simulink model "volt_mfile"  (R2019a)
settings: Solver=VariableStepAuto  StartTime=0.0  StopTime=5  RelTol=1e-3
settings Model: Creator=USER  LastModifiedBy=USER

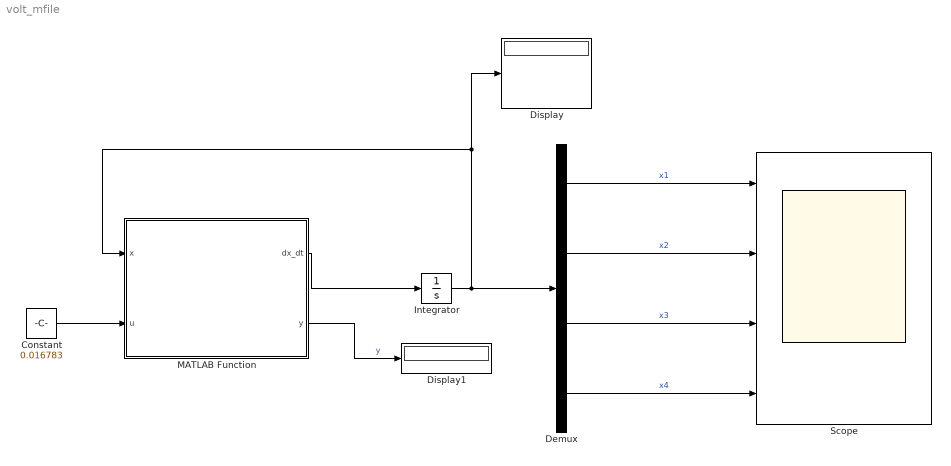
== system volt_mfile ==
  Constant : Constant  Value=0.016783
  Demux : Demux
  Display : Display
  Display1 : Display
  Integrator : Integrator  InitialCondition=[6,8,0,0]
  MATLAB Function : MATLAB Function  TreatAsAtomicUnit=on
  Scope : Scope  NumInputPorts=4
  wires:
  MATLAB Function/1(dx_dt) -> Integrator/1
  Integrator/1 -> MATLAB Function/1(x), Display/1, Demux/1
  Constant/1 -> MATLAB Function/2(u)
  Demux/1 -> Scope/1  "x1"
  Demux/2 -> Scope/2  "x2"
  Demux/3 -> Scope/3  "x3"
  Demux/4 -> Scope/4  "x4"
  MATLAB Function/2(y) -> Display1/1  "y"

== matlab function volt_mfile/MATLAB Function ==
  data: x input; u input; dx_dt output; y output
function [dx_dt, y] = volt(x,u)
% defining the parameters


%outputs
Cm = x(1);
Ci = x(2);
Do = x(3);
Di = x(4);
y = Di/Do;

%inputs
u = u(1);

%initialize the differential equations
dx_dt = zeros(4,1);

%defining the differential equations

dx_dt(1) = 10*(6-Cm) - (2.4568*Cm*sqrt(Ci)); 
 
dx_dt(2) = 80*u - 10.1022*Ci;
 
dx_dt(3) = 0.0024121*Cm*sqrt(Ci) + 0.112191*Ci - 10*Do;
 
dx_dt(4) = 245.978*Cm*sqrt(Ci) - 10*Di;
